simulink model "planta"  (Simulink 9.0)
settings: Solver=ode45  StartTime=0.0  StopTime=100  RelTol=1e-3  EnableMultiTasking=on
libraries: simulink x3
settings Model: Creator=juan  LastModifiedBy=usuario_local  ExtModeAutoUpdateStatusClock=off
settings DataIOCC: LimitDataPoints=on  SignalLoggingSaveFormat=ModelDataLogs
settings OptimizationCC: InitFltsAndDblsToZero=on
settings DebuggingCC: SaveWithParameterizedLinksMsg=none  SignalResolutionControl=TryResolveAllWithWarning  SolverPrmCheckMsg=warning  FcnCallInpInsideContextMsg=warning  StrictBusMsg=Warning
settings GRTTargetCC: TargetFcnLib=ansi_tfl_tmw.mat  CombineOutputUpdateFcns=off  GRTInterface=on

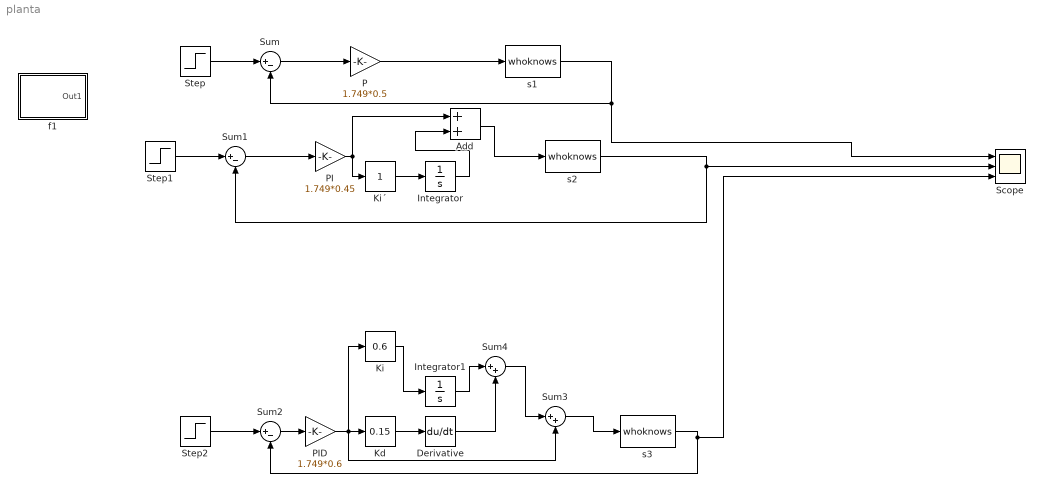
== system planta ==
  Add : Sum
  Derivative : Derivative
  Integrator : Integrator
  Integrator1 : Integrator
  Kd : simulink/Math Operations/Slider Gain  gain=0.15  low=0  high=2
  Ki : simulink/Math Operations/Slider Gain  gain=0.6  low=0  high=2
  Ki´ : simulink/Math Operations/Slider Gain  gain=1  low=0  high=2
  P : Gain  Gain=1.749*0.5
  PI : Gain  Gain=1.749*0.45
  PID : Gain  Gain=1.749*0.6
  Scope : Scope  NumInputPorts=3
  Step : Step  SampleTime=0
  Step1 : Step  SampleTime=0
  Step2 : Step  SampleTime=0
  Sum : Sum  Inputs=|+-
  Sum1 : Sum  Inputs=|+-
  Sum2 : Sum  Inputs=|+-
  Sum3 : Sum  Inputs=|++
  Sum4 : Sum  Inputs=|++
  f1 : Subsystem  mask{S=1, L=0, T=2}
      mask prompts: S "Limite Superior"; L "Limite Inferior"; T "Periodo de cambio"
      mask Display: disp('Ent. Variable')
  s1 : M-S-Function  FunctionName=whoknows  Parameters=L, P1, P2, T, R  mask{L=7, P1=0, P2=6, T=2, R=0}
      mask prompts: L "Laboratorio"; P1 "Primer digito del Puesto"; P2 "Segundo digito del Puesto"; T "Tipo de Planta"; R "Ruido"
      mask Display: disp('Sistema')
  s2 : M-S-Function  FunctionName=whoknows  Parameters=L, P1, P2, T, R  mask{L=7, P1=0, P2=6, T=2, R=0}
      mask prompts: L "Laboratorio"; P1 "Primer digito del Puesto"; P2 "Segundo digito del Puesto"; T "Tipo de Planta"; R "Ruido"
      mask Display: disp('Sistema')
  s3 : M-S-Function  FunctionName=whoknows  Parameters=L, P1, P2, T, R  mask{L=7, P1=0, P2=6, T=2, R=0}
      mask prompts: L "Laboratorio"; P1 "Primer digito del Puesto"; P2 "Segundo digito del Puesto"; T "Tipo de Planta"; R "Ruido"
      mask Display: disp('Sistema')
  wires:
  Step/1 -> Sum/1
  Sum/1 -> P/1
  P/1 -> s1/1
  s1/1 -> Sum/2, Scope/1
  s2/1 -> Scope/2, Sum1/2
  Sum1/1 -> PI/1
  Step1/1 -> Sum1/1
  s3/1 -> Scope/3, Sum2/2
  Sum2/1 -> PID/1
  Step2/1 -> Sum2/1
  Derivative/1 -> Sum4/2
  PID/1 -> Kd/1, Sum3/2, Ki/1
  PI/1 -> Add/1, Ki´/1
  Integrator/1 -> Add/2
  Add/1 -> s2/1
  Sum3/1 -> s3/1
  Sum4/1 -> Sum3/1
  Integrator1/1 -> Sum4/1
  Ki´/1 -> Integrator/1
  Ki/1 -> Integrator1/1
  Kd/1 -> Derivative/1

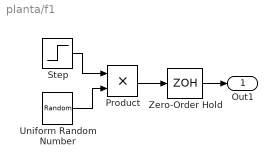
== system planta/f1 ==
  Product : Product  RndMeth=Zero
  Step : Step  Time=0  SampleTime=0
  Uniform Random Number : UniformRandomNumber  Minimum=L  Maximum=S  SampleTime=0
  Zero-Order Hold : ZeroOrderHold  SampleTime=T
  Out1 : Outport
  wires:
  Step/1 -> Product/1
  Uniform Random Number/1 -> Product/2
  Product/1 -> Zero-Order Hold/1
  Zero-Order Hold/1 -> Out1/1
